simulink model "Pix_FCC_flash"  (R2019b)
settings: Solver=FixedStepAuto  StartTime=0.0  StopTime=inf  RelTol=1e-3  EnableMultiTasking=on
undefined symbols (not defined in the file or in its folder): dev, FCC_PIX_Data, Main, pwm_output0
libraries: px4lib x14, simulink x10, px4Sensorslib x3
(part 2 of 2)

== matlab function Pix_FCC_flash/ExecutionCycle/process_received_data/input_hold/ByteUnpack ==
  data: message input uint8 size=[1 56]; SimHeartbeat output uint16 size=1; SimStatus output; SimRCStatus output; CMD output single size=3; ACC output single size=3; ROT output single size=3; ATT output single size=[1 3]; TestSignal output single size=1
function [SimHeartbeat,SimStatus,SimRCStatus,CMD,ACC,ROT,ATT,TestSignal] = ByteUnpack(message)
    
    %specify size and type of input and output data in data manager!!
    
    SimHeartbeat = typecast(uint8(message(1:2)),'uint16');
    SimStatus = message(3);
    SimRCStatus = message(4);
    
    CMD1 = typecast(uint8(message(5:8)),'single');
    CMD2 = typecast(uint8(message(9:12)),'single');
    CMD3 = typecast(uint8(message(13:16)),'single');
    CMD = [CMD1 CMD2 CMD3]';
    
    ACC1 = typecast(uint8(message(17:20)),'single');
    ACC2 = typecast(uint8(message(21:24)),'single');
    ACC3 = typecast(uint8(message(25:28)),'single');
    ACC = [ACC1 ACC2 ACC3]';
    
    ROT1 = typecast(uint8(message(29:32)),'single');
    ROT2 = typecast(uint8(message(33:36)),'single');
    ROT3 = typecast(uint8(message(37:40)),'single');
    ROT = [ROT1 ROT2 ROT3]';
    
    ATT_phi = typecast(uint8(message(41:44)),'single');
    ATT_theta = typecast(uint8(message(45:48)),'single');
    ATT_psi = typecast(uint8(message(49:52)),'single');
    ATT = [ATT_phi ATT_theta ATT_psi];
    
    TestSignal = typecast(uint8(message(53:56)),'single');
    
end

== matlab function Pix_FCC_flash/ExecutionCycle/OUTPUT/serial send/MessageAssembly_Complete ==
  data: SendingMode input double size=1; MessageToSend output uint8 size=[1 58]; PixHeartbeat input uint16 size=1; PixStatus input uint8 size=1; RCStatus input uint8 size=1; DataToSend input single size=[10 1]
function MessageToSend = MessageAssembly(SendingMode, PixHeartbeat, PixStatus, RCStatus, DataToSend)
    
    
    %specify size and type of input and output data in data manager!!
    
    if SendingMode == 1
        
        DataToSend = DataToSend';
        
        whiteNoise = uint8([0 0 0 0 0]);
        
        package = [typecast(uint16(PixHeartbeat),'uint8') PixStatus RCStatus typecast(single(DataToSend),'uint8')];
        
        headerToSend = uint8([5 5]);
        packetToSend = uint8(package);
        
        MessageToSend = [whiteNoise headerToSend packetToSend headerToSend whiteNoise];
        
        %fwrite(s,dataToSend);
        %bytes_sent = s.ValuesSent;
        
    else
        
        MessageToSend = uint8(zeros(1,58));
        
    end
    
    
end

== matlab function Pix_FCC_flash/Command_Chain/SetMode ==
  data: cmd input uint8 size=[4 1]; mode output double size=1; HIL_flg input boolean size=1
function mode = SetMode(cmd,HIL_flg)
    
    % adapt!!!! TBD!!!
    
    mode = 1; %default option
    
    cmd_mode = cmd(1);
    cmd_rate = cmd(2);
    cmd_com_rate = cmd(3);
    cmd_default = cmd(4);
    
    if HIL_flg %in HIL mode % TBD!!!
        
        switch cmd_mode
            case 1
                mode = 2;
            case 2
                mode = 3;
            case 3
                mode = 4;
        end
        
        % extend to support different sample rates for the execution cycle
        % and the communication for every mode!!
        
    else %real flight
        
        mode = 1;
        
    end
        
    
end

== matlab function Pix_FCC_flash/Command_Chain/DecodeCommand/DecodeCommand ==
  data: message input uint8 size=[128 1]; cmd output uint8 size=[4 1]; cmd_found_flg output boolean size=1
function [cmd,cmd_found_flg] = DecodeCommand(message)
    
    %specify size and type of input and output data in data manager!!
    
    message = message';
    expected_message_length = 4; % specify!!
    expected_header = [8 8];      % specify!!
    expected_header_length = length(expected_header);
    expected_packet_length = expected_message_length + expected_header_length;
    
    packet = uint8(zeros(1,expected_message_length));
    cmd_found_flg = false;
    
    %% locate packet in data
    
    % First, find possible header start locations; i.e., match the first element in the
    % header.
    start = find(message==expected_header(1));
    
    % Next remove start values that are too close to the end to possibly match
    % the header.
    endVals = start+expected_header_length-1;
    start(endVals>length(message)) = [];
    
    % Next, loop over elements of header, usually much shorter than length of
    % array, to check which possible header start locations are valid still.
    for pattval = 2:expected_header_length
        % check viable locations in array
        locs = expected_header(pattval) == message(start+pattval-1);
        % delete false ones from indices
        start(~locs) = [];
    end
    
    %Packet = Data - Header
    if ~isempty(start)
        for i = 1:(length(start)-1)
            %Verify if the size of data between 2 consecutive header start
            %indices is equal to the expectedPacketSize
            if isequal(start(i+1)-start(i),expected_packet_length)
            
                %Extract the packet by stripping the header from the data
                packet = message(start(i)+expected_header_length:start(i+1)-1);
                if ~isequal(length(packet),(expected_packet_length-expected_header_length))
                    error('ERROR:Wrong packet size');
                end
            
                %Once a valid packet is found, exit the for loop
                cmd_found_flg = true;
                break;
            else
                continue
            end
        end
    else
        cmd_found_flg = false;
        packet = uint8([0 0 0 0]);
    end
    
    
    
    %% extract command
    
    cmd = uint8(packet);
    
    
    
    
    
    
    
    
end

== matlab function Pix_FCC_flash/Synchronisation/ControlExecution ==
  data: mode input; enable_execution output; status input; enable_trigger_inh output; enable_trigger_10Hz output; enable_trigger_100Hz output
function [enable_execution, enable_trigger_inh, enable_trigger_10Hz, enable_trigger_100Hz] = ControlExecution(mode,status)
    
    switch mode
        case 1
            enable_execution = 1;
            enable_trigger_inh = 0;
            enable_trigger_10Hz = 0;
            enable_trigger_100Hz = 1;
        case 2
            enable_execution = double(status);
            enable_trigger_inh = 1;
            enable_trigger_10Hz = 0;
            enable_trigger_100Hz = 0;
        case 3
            enable_execution = 1;
            enable_trigger_inh = 0;
            enable_trigger_10Hz = 0;
            enable_trigger_100Hz = 1;
        case 4
            enable_execution = 1;
            enable_trigger_inh = 0;
            enable_trigger_10Hz = 0;
            enable_trigger_100Hz = 1;
        otherwise
            enable_execution = 1;
            enable_trigger_inh = 0;
            enable_trigger_10Hz = 0;
            enable_trigger_100Hz = 1;
    end
    
    
end

== matlab function Pix_FCC_flash/ExecutionCycle/ACTION/DefineStatus ==
  data: mode input; PixStatus output
function PixStatus = DefineStatus(mode)
    
    %extend??!
    PixStatus = uint8(mode);
    
end

== matlab function Pix_FCC_flash/ExecutionCycle/ACTION/DefineRCStatus ==
  data: packetfound_flg input; RCStatus output
function RCStatus = DefineRCStatus(packetfound_flg)
    
    %maybe also include if data was received or not??!
    
    RCStatus = uint8(packetfound_flg);
    
end

== matlab function Pix_FCC_flash/Command_Chain/DecodeCommand/ConfirmCommand/pack ==
  data: in input uint8 size=[4 1]; send output single size=1
function send = pack(in)
    
    pack = [uint8(in(1)) uint8(in(2)) uint8(in(3)) uint8(in(4))];
    send = typecast(uint8(pack),'single');
    
end
